simulink model "prob_6"  (R2020b)
settings: Solver=VariableStepAuto  StartTime=0.0  StopTime=10.0  RelTol=1e-3
settings Model: Creator=nadee  LastModifiedBy=nadee

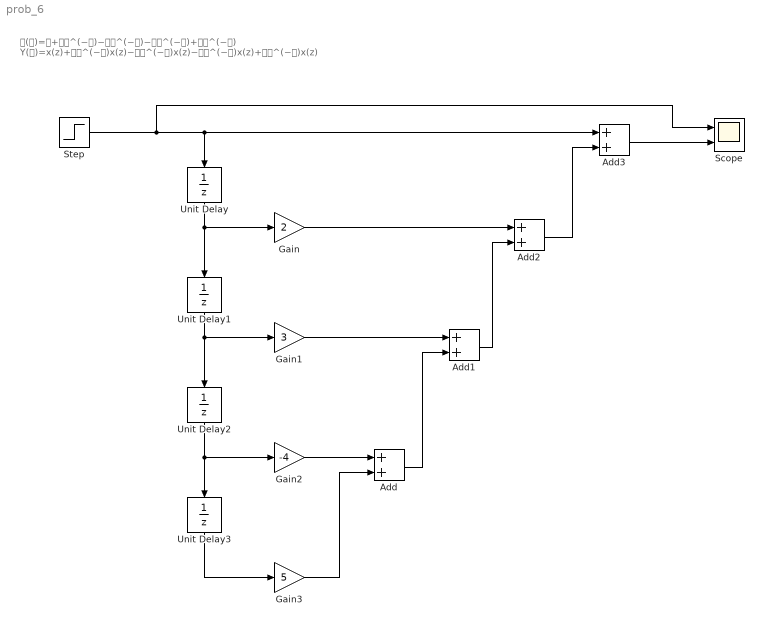
== system prob_6 ==
  note: 𝐇(𝐳)=𝟏+𝟐𝐳^(−𝟏)−𝟑𝐳^(−𝟐)−𝟒𝐳^(−𝟑)+𝟓𝐳^(−𝟒)
      | Y(𝐳)=x(z)+𝟐𝐳^(−𝟏)x(z)−𝟑𝐳^(−𝟐)x(z)−𝟒𝐳^(−𝟑)x(z)+𝟓𝐳^(−𝟒)x(z)
  Add{,1..3} (4 alike) : Sum
  Gain : Gain  Gain=2
  Gain1 : Gain  Gain=3
  Gain2 : Gain  Gain=-4
  Gain3 : Gain  Gain=5
  Scope : Scope  NumInputPorts=2
  Step : Step  SampleTime=0
  Unit Delay{,1..3} (4 alike) : UnitDelay  SampleTime=-1  HasFrameUpgradeWarning=on
  wires:
  Gain2/1 -> Add/1
  Gain3/1 -> Add/2
  Add/1 -> Add1/2
  Add1/1 -> Add2/2
  Add2/1 -> Add3/2
  Unit Delay3/1 -> Gain3/1
  Unit Delay2/1 -> Gain2/1, Unit Delay3/1
  Unit Delay1/1 -> Unit Delay2/1, Gain1/1
  Gain1/1 -> Add1/1
  Gain/1 -> Add2/1
  Unit Delay/1 -> Gain/1, Unit Delay1/1
  Step/1 -> Unit Delay/1, Add3/1, Scope/1
  Add3/1 -> Scope/2
